simulink model "Oscillator_Sync_Aperiodic"  (Simulink 10.0)
settings: Solver=ode45  StartTime=0.0  StopTime=T  MaxStep=MaxStep  RelTol=RelTol  EnableMultiTasking=on
values from neighbouring files (symbols this model uses):
  J = 30    [initialization_Oscillator_Sync_Aperiodic.m]
  Kmatrix = [-1 -2]    [initialization_Oscillator_Sync_Aperiodic.m]
  rule = 1    [initialization_Oscillator_Sync_Aperiodic.m]
  T = 15    [initialization_Oscillator_Sync_Aperiodic.m]
undefined symbols (not defined in the file): x11_0, x1_0, x22_0, x2_0, x33_0, x3_0, x44_0, x4_0
libraries: simulink x24, HyEQ_Library_R2012a x2
(part 2 of 2)

== system Oscillator_Sync_Aperiodic/Aperiodic Sampling 4/Integrator System/Jump logic ==
  note: rule=1:  out = D
      | rlule=2: out = D and ~C
      | rule=3:  out = (D and ~C)  or (D and C and r>0.5)
      | other :  out = 0
  C : Inport
  D : Inport  Port=2
  r : Inport  Port=3
  Compare To Constant : simulink/Logic and Bit Operations/Compare To Constant  relop=>=  const=0.5  OutDataTypeStr=uint8
  Constant : Constant  Value=rule
  Logical Operator : Logic  AllPortsSameDT=off  OutDataTypeStr=boolean
  Logical Operator1 : Logic  Operator=NOT  Inputs=1  AllPortsSameDT=off  OutDataTypeStr=boolean
  Logical Operator2 : Logic  Operator=OR  AllPortsSameDT=off  OutDataTypeStr=boolean
  Logical Operator3 : Logic  Inputs=3  AllPortsSameDT=off  OutDataTypeStr=boolean
  Multiport Switch : MultiPortSwitch
  jump : Outport
  wires:
  Logical Operator3/1 -> Logical Operator2/2
  Compare To Constant/1 -> Logical Operator3/3
  Multiport Switch/1 -> jump/1
  Logical Operator2/1 -> Multiport Switch/4
  Logical Operator/1 -> Logical Operator2/1, Multiport Switch/3
  Logical Operator1/1 -> Logical Operator/2
  C/1 -> Logical Operator1/1, Logical Operator3/2
  r/1 -> Compare To Constant/1
  D/1 -> Multiport Switch/2, Logical Operator/1, Logical Operator3/1
  Constant/1 -> Multiport Switch/1

== system Oscillator_Sync_Aperiodic/Aperiodic Sampling 4/Integrator System/Stop logic ==
  t : Inport
  j : Inport  Port=2
  C : Inport  Port=3
  D : Inport  Port=4
  "Flow Horizon, T" : simulink/Logic and Bit Operations/Compare To Constant  relop=>=  const=T  OutDataTypeStr=uint8  ZeroCross=off
  "Jump Horizon, J" : simulink/Logic and Bit Operations/Compare To Constant  relop=>=  const=J  OutDataTypeStr=uint8  ZeroCross=off
  Logical Operator : Logic  Operator=NOR  AllPortsSameDT=off  OutDataTypeStr=boolean
  Logical Operator1 : Logic  Operator=OR  Inputs=3  AllPortsSameDT=off  OutDataTypeStr=boolean
  stop : Outport
  wires:
  Logical Operator1/1 -> stop/1
  C/1 -> Logical Operator/1
  j/1 -> "Jump Horizon, J"/1
  t/1 -> "Flow Horizon, T"/1
  D/1 -> Logical Operator/2
  Logical Operator/1 -> Logical Operator1/3
  "Jump Horizon, J"/1 -> Logical Operator1/2
  "Flow Horizon, T"/1 -> Logical Operator1/1

== system Oscillator_Sync_Aperiodic/Aperiodic Sampling 4/Integrator System/Update logic ==
  g(x-,u) : Inport
  j- : Inport  Port=2
  t- : Inport  Port=3
  Constant : Constant
  Mux1 : Mux  Inputs=[1 1 -1]
  Sum : Sum  Inputs=|++
  update law : Outport
  wires:
  Constant/1 -> Sum/2
  t-/1 -> Mux1/1
  g(x-,u)/1 -> Mux1/3
  j-/1 -> Sum/1
  Mux1/1 -> update law/1
  Sum/1 -> Mux1/2

== system Oscillator_Sync_Aperiodic/Oscillator 1/Integrator System/CT dynamics ==
  f(x,u) : Inport
  Flows : Constant
  Jumps : Constant  Value=0
  Mux : Mux  Inputs=[1 1 -1]
  dot : Outport
  wires:
  f(x,u)/1 -> Mux/3
  Mux/1 -> dot/1
  Flows/1 -> Mux/1
  Jumps/1 -> Mux/2

== system Oscillator_Sync_Aperiodic/Oscillator 1/Integrator System/Jump logic ==
  note: rule=1:  out = D
      | rlule=2: out = D and ~C
      | rule=3:  out = (D and ~C)  or (D and C and r>0.5)
      | other :  out = 0
  C : Inport
  D : Inport  Port=2
  r : Inport  Port=3
  Compare To Constant : simulink/Logic and Bit Operations/Compare To Constant  relop=>=  const=0.5  OutDataTypeStr=uint8
  Constant : Constant  Value=rule
  Logical Operator : Logic  AllPortsSameDT=off  OutDataTypeStr=boolean
  Logical Operator1 : Logic  Operator=NOT  Inputs=1  AllPortsSameDT=off  OutDataTypeStr=boolean
  Logical Operator2 : Logic  Operator=OR  AllPortsSameDT=off  OutDataTypeStr=boolean
  Logical Operator3 : Logic  Inputs=3  AllPortsSameDT=off  OutDataTypeStr=boolean
  Multiport Switch : MultiPortSwitch
  jump : Outport
  wires:
  Logical Operator3/1 -> Logical Operator2/2
  Compare To Constant/1 -> Logical Operator3/3
  Multiport Switch/1 -> jump/1
  Logical Operator2/1 -> Multiport Switch/4
  Logical Operator/1 -> Logical Operator2/1, Multiport Switch/3
  Logical Operator1/1 -> Logical Operator/2
  C/1 -> Logical Operator1/1, Logical Operator3/2
  r/1 -> Compare To Constant/1
  D/1 -> Multiport Switch/2, Logical Operator/1, Logical Operator3/1
  Constant/1 -> Multiport Switch/1

== system Oscillator_Sync_Aperiodic/Oscillator 1/Integrator System/Stop logic ==
  t : Inport
  j : Inport  Port=2
  C : Inport  Port=3
  D : Inport  Port=4
  "Flow Horizon, T" : simulink/Logic and Bit Operations/Compare To Constant  relop=>=  const=T  OutDataTypeStr=uint8  ZeroCross=off
  "Jump Horizon, J" : simulink/Logic and Bit Operations/Compare To Constant  relop=>=  const=J  OutDataTypeStr=uint8  ZeroCross=off
  Logical Operator : Logic  Operator=NOR  AllPortsSameDT=off  OutDataTypeStr=boolean
  Logical Operator1 : Logic  Operator=OR  Inputs=3  AllPortsSameDT=off  OutDataTypeStr=boolean
  stop : Outport
  wires:
  Logical Operator1/1 -> stop/1
  C/1 -> Logical Operator/1
  j/1 -> "Jump Horizon, J"/1
  t/1 -> "Flow Horizon, T"/1
  D/1 -> Logical Operator/2
  Logical Operator/1 -> Logical Operator1/3
  "Jump Horizon, J"/1 -> Logical Operator1/2
  "Flow Horizon, T"/1 -> Logical Operator1/1

== system Oscillator_Sync_Aperiodic/Oscillator 1/Integrator System/Update logic ==
  g(x-,u) : Inport
  j- : Inport  Port=2
  t- : Inport  Port=3
  Constant : Constant
  Mux1 : Mux  Inputs=[1 1 -1]
  Sum : Sum  Inputs=|++
  update law : Outport
  wires:
  Constant/1 -> Sum/2
  t-/1 -> Mux1/1
  g(x-,u)/1 -> Mux1/3
  j-/1 -> Sum/1
  Mux1/1 -> update law/1
  Sum/1 -> Mux1/2

== system Oscillator_Sync_Aperiodic/Oscillator 2/Integrator System/CT dynamics ==
  f(x,u) : Inport
  Flows : Constant
  Jumps : Constant  Value=0
  Mux : Mux  Inputs=[1 1 -1]
  dot : Outport
  wires:
  f(x,u)/1 -> Mux/3
  Mux/1 -> dot/1
  Flows/1 -> Mux/1
  Jumps/1 -> Mux/2

== system Oscillator_Sync_Aperiodic/Oscillator 2/Integrator System/Jump logic ==
  note: rule=1:  out = D
      | rlule=2: out = D and ~C
      | rule=3:  out = (D and ~C)  or (D and C and r>0.5)
      | other :  out = 0
  C : Inport
  D : Inport  Port=2
  r : Inport  Port=3
  Compare To Constant : simulink/Logic and Bit Operations/Compare To Constant  relop=>=  const=0.5  OutDataTypeStr=uint8
  Constant : Constant  Value=rule
  Logical Operator : Logic  AllPortsSameDT=off  OutDataTypeStr=boolean
  Logical Operator1 : Logic  Operator=NOT  Inputs=1  AllPortsSameDT=off  OutDataTypeStr=boolean
  Logical Operator2 : Logic  Operator=OR  AllPortsSameDT=off  OutDataTypeStr=boolean
  Logical Operator3 : Logic  Inputs=3  AllPortsSameDT=off  OutDataTypeStr=boolean
  Multiport Switch : MultiPortSwitch
  jump : Outport
  wires:
  Logical Operator3/1 -> Logical Operator2/2
  Compare To Constant/1 -> Logical Operator3/3
  Multiport Switch/1 -> jump/1
  Logical Operator2/1 -> Multiport Switch/4
  Logical Operator/1 -> Logical Operator2/1, Multiport Switch/3
  Logical Operator1/1 -> Logical Operator/2
  C/1 -> Logical Operator1/1, Logical Operator3/2
  r/1 -> Compare To Constant/1
  D/1 -> Multiport Switch/2, Logical Operator/1, Logical Operator3/1
  Constant/1 -> Multiport Switch/1

== system Oscillator_Sync_Aperiodic/Oscillator 2/Integrator System/Stop logic ==
  t : Inport
  j : Inport  Port=2
  C : Inport  Port=3
  D : Inport  Port=4
  "Flow Horizon, T" : simulink/Logic and Bit Operations/Compare To Constant  relop=>=  const=T  OutDataTypeStr=uint8  ZeroCross=off
  "Jump Horizon, J" : simulink/Logic and Bit Operations/Compare To Constant  relop=>=  const=J  OutDataTypeStr=uint8  ZeroCross=off
  Logical Operator : Logic  Operator=NOR  AllPortsSameDT=off  OutDataTypeStr=boolean
  Logical Operator1 : Logic  Operator=OR  Inputs=3  AllPortsSameDT=off  OutDataTypeStr=boolean
  stop : Outport
  wires:
  Logical Operator1/1 -> stop/1
  C/1 -> Logical Operator/1
  j/1 -> "Jump Horizon, J"/1
  t/1 -> "Flow Horizon, T"/1
  D/1 -> Logical Operator/2
  Logical Operator/1 -> Logical Operator1/3
  "Jump Horizon, J"/1 -> Logical Operator1/2
  "Flow Horizon, T"/1 -> Logical Operator1/1

== system Oscillator_Sync_Aperiodic/Oscillator 2/Integrator System/Update logic ==
  g(x-,u) : Inport
  j- : Inport  Port=2
  t- : Inport  Port=3
  Constant : Constant
  Mux1 : Mux  Inputs=[1 1 -1]
  Sum : Sum  Inputs=|++
  update law : Outport
  wires:
  Constant/1 -> Sum/2
  t-/1 -> Mux1/1
  g(x-,u)/1 -> Mux1/3
  j-/1 -> Sum/1
  Mux1/1 -> update law/1
  Sum/1 -> Mux1/2

== system Oscillator_Sync_Aperiodic/Oscillator 3/Integrator System/CT dynamics ==
  f(x,u) : Inport
  Flows : Constant
  Jumps : Constant  Value=0
  Mux : Mux  Inputs=[1 1 -1]
  dot : Outport
  wires:
  f(x,u)/1 -> Mux/3
  Mux/1 -> dot/1
  Flows/1 -> Mux/1
  Jumps/1 -> Mux/2

== system Oscillator_Sync_Aperiodic/Oscillator 3/Integrator System/Jump logic ==
  note: rule=1:  out = D
      | rlule=2: out = D and ~C
      | rule=3:  out = (D and ~C)  or (D and C and r>0.5)
      | other :  out = 0
  C : Inport
  D : Inport  Port=2
  r : Inport  Port=3
  Compare To Constant : simulink/Logic and Bit Operations/Compare To Constant  relop=>=  const=0.5  OutDataTypeStr=uint8
  Constant : Constant  Value=rule
  Logical Operator : Logic  AllPortsSameDT=off  OutDataTypeStr=boolean
  Logical Operator1 : Logic  Operator=NOT  Inputs=1  AllPortsSameDT=off  OutDataTypeStr=boolean
  Logical Operator2 : Logic  Operator=OR  AllPortsSameDT=off  OutDataTypeStr=boolean
  Logical Operator3 : Logic  Inputs=3  AllPortsSameDT=off  OutDataTypeStr=boolean
  Multiport Switch : MultiPortSwitch
  jump : Outport
  wires:
  Logical Operator3/1 -> Logical Operator2/2
  Compare To Constant/1 -> Logical Operator3/3
  Multiport Switch/1 -> jump/1
  Logical Operator2/1 -> Multiport Switch/4
  Logical Operator/1 -> Logical Operator2/1, Multiport Switch/3
  Logical Operator1/1 -> Logical Operator/2
  C/1 -> Logical Operator1/1, Logical Operator3/2
  r/1 -> Compare To Constant/1
  D/1 -> Multiport Switch/2, Logical Operator/1, Logical Operator3/1
  Constant/1 -> Multiport Switch/1

== system Oscillator_Sync_Aperiodic/Oscillator 3/Integrator System/Stop logic ==
  t : Inport
  j : Inport  Port=2
  C : Inport  Port=3
  D : Inport  Port=4
  "Flow Horizon, T" : simulink/Logic and Bit Operations/Compare To Constant  relop=>=  const=T  OutDataTypeStr=uint8  ZeroCross=off
  "Jump Horizon, J" : simulink/Logic and Bit Operations/Compare To Constant  relop=>=  const=J  OutDataTypeStr=uint8  ZeroCross=off
  Logical Operator : Logic  Operator=NOR  AllPortsSameDT=off  OutDataTypeStr=boolean
  Logical Operator1 : Logic  Operator=OR  Inputs=3  AllPortsSameDT=off  OutDataTypeStr=boolean
  stop : Outport
  wires:
  Logical Operator1/1 -> stop/1
  C/1 -> Logical Operator/1
  j/1 -> "Jump Horizon, J"/1
  t/1 -> "Flow Horizon, T"/1
  D/1 -> Logical Operator/2
  Logical Operator/1 -> Logical Operator1/3
  "Jump Horizon, J"/1 -> Logical Operator1/2
  "Flow Horizon, T"/1 -> Logical Operator1/1

== system Oscillator_Sync_Aperiodic/Oscillator 3/Integrator System/Update logic ==
  g(x-,u) : Inport
  j- : Inport  Port=2
  t- : Inport  Port=3
  Constant : Constant
  Mux1 : Mux  Inputs=[1 1 -1]
  Sum : Sum  Inputs=|++
  update law : Outport
  wires:
  Constant/1 -> Sum/2
  t-/1 -> Mux1/1
  g(x-,u)/1 -> Mux1/3
  j-/1 -> Sum/1
  Mux1/1 -> update law/1
  Sum/1 -> Mux1/2

== system Oscillator_Sync_Aperiodic/Oscillator 4/Integrator System/CT dynamics ==
  f(x,u) : Inport
  Flows : Constant
  Jumps : Constant  Value=0
  Mux : Mux  Inputs=[1 1 -1]
  dot : Outport
  wires:
  f(x,u)/1 -> Mux/3
  Mux/1 -> dot/1
  Flows/1 -> Mux/1
  Jumps/1 -> Mux/2

== system Oscillator_Sync_Aperiodic/Oscillator 4/Integrator System/Jump logic ==
  note: rule=1:  out = D
      | rlule=2: out = D and ~C
      | rule=3:  out = (D and ~C)  or (D and C and r>0.5)
      | other :  out = 0
  C : Inport
  D : Inport  Port=2
  r : Inport  Port=3
  Compare To Constant : simulink/Logic and Bit Operations/Compare To Constant  relop=>=  const=0.5  OutDataTypeStr=uint8
  Constant : Constant  Value=rule
  Logical Operator : Logic  AllPortsSameDT=off  OutDataTypeStr=boolean
  Logical Operator1 : Logic  Operator=NOT  Inputs=1  AllPortsSameDT=off  OutDataTypeStr=boolean
  Logical Operator2 : Logic  Operator=OR  AllPortsSameDT=off  OutDataTypeStr=boolean
  Logical Operator3 : Logic  Inputs=3  AllPortsSameDT=off  OutDataTypeStr=boolean
  Multiport Switch : MultiPortSwitch
  jump : Outport
  wires:
  Logical Operator3/1 -> Logical Operator2/2
  Compare To Constant/1 -> Logical Operator3/3
  Multiport Switch/1 -> jump/1
  Logical Operator2/1 -> Multiport Switch/4
  Logical Operator/1 -> Logical Operator2/1, Multiport Switch/3
  Logical Operator1/1 -> Logical Operator/2
  C/1 -> Logical Operator1/1, Logical Operator3/2
  r/1 -> Compare To Constant/1
  D/1 -> Multiport Switch/2, Logical Operator/1, Logical Operator3/1
  Constant/1 -> Multiport Switch/1

== system Oscillator_Sync_Aperiodic/Oscillator 4/Integrator System/Stop logic ==
  t : Inport
  j : Inport  Port=2
  C : Inport  Port=3
  D : Inport  Port=4
  "Flow Horizon, T" : simulink/Logic and Bit Operations/Compare To Constant  relop=>=  const=T  OutDataTypeStr=uint8  ZeroCross=off
  "Jump Horizon, J" : simulink/Logic and Bit Operations/Compare To Constant  relop=>=  const=J  OutDataTypeStr=uint8  ZeroCross=off
  Logical Operator : Logic  Operator=NOR  AllPortsSameDT=off  OutDataTypeStr=boolean
  Logical Operator1 : Logic  Operator=OR  Inputs=3  AllPortsSameDT=off  OutDataTypeStr=boolean
  stop : Outport
  wires:
  Logical Operator1/1 -> stop/1
  C/1 -> Logical Operator/1
  j/1 -> "Jump Horizon, J"/1
  t/1 -> "Flow Horizon, T"/1
  D/1 -> Logical Operator/2
  Logical Operator/1 -> Logical Operator1/3
  "Jump Horizon, J"/1 -> Logical Operator1/2
  "Flow Horizon, T"/1 -> Logical Operator1/1

== system Oscillator_Sync_Aperiodic/Oscillator 4/Integrator System/Update logic ==
  g(x-,u) : Inport
  j- : Inport  Port=2
  t- : Inport  Port=3
  Constant : Constant
  Mux1 : Mux  Inputs=[1 1 -1]
  Sum : Sum  Inputs=|++
  update law : Outport
  wires:
  Constant/1 -> Sum/2
  t-/1 -> Mux1/1
  g(x-,u)/1 -> Mux1/3
  j-/1 -> Sum/1
  Mux1/1 -> update law/1
  Sum/1 -> Mux1/2

== matlab function Oscillator 1/flow map f ==
  data: tau input double; taudot output double; u input double
function taudot = f(tau, u)

%%%%%%%%%%%%%%%%%%%%%%%%%%%%%%%%%%%%%%%%%%%%%%%%%%%%%%%%%%%%%%%%%%%%%%%%%%%
% Matlab Function  Author: Ricardo Sanfelice
%
% Project: Simulation of a hybrid system (interconnection)
%
% Name: f.m
%
% Description: Flow map
%
% Version: 1.0
% Required files: - 
%%%%%%%%%%%%%%%%%%%%%%%%%%%%%%%%%%%%%%%%%%%%%%%%%%%%%%%%%%%%%%%%%%%%%%%%%%%

% flow map
Amatrix = [0 1;-1 0];
Bmatrix = [0;1];
taudot = Amatrix*tau + Bmatrix*u;

== matlab function Oscillator 1/flow set C ==
  data: tau input double; v output double; u input double
function v  = C(tau, u) 

%%%%%%%%%%%%%%%%%%%%%%%%%%%%%%%%%%%%%%%%%%%%%%%%%%%%%%%%%%%%%%%%%%%%%%%%%%%
% Matlab Function  Author: Ricardo Sanfelice 
%
% Project: Simulation of a hybrid system (interconnection)
%
% Name: C.m
%
% Description: Flow set
%
% Version: 1.0
% Required files: - 
%%%%%%%%%%%%%%%%%%%%%%%%%%%%%%%%%%%%%%%%%%%%%%%%%%%%%%%%%%%%%%%%%%%%%%%%%%%

%flow set
% if ((tau > 0) && (tau < 1)) || ((u > 0) && (u <= 1))  % flow condition
%     v = 1;  % report flow
% else 
%     v = 0;  % do not report flow
% end
v = 1;

== matlab function Oscillator 2/flow map f ==
  data: tau input double; taudot output double; u input double
function taudot = f(tau, u)

%%%%%%%%%%%%%%%%%%%%%%%%%%%%%%%%%%%%%%%%%%%%%%%%%%%%%%%%%%%%%%%%%%%%%%%%%%%
% Matlab Function  Author: Ricardo Sanfelice
%
% Project: Simulation of a hybrid system (interconnection)
%
% Name: f.m
%
% Description: Flow map
%
% Version: 1.0
% Required files: - 
%%%%%%%%%%%%%%%%%%%%%%%%%%%%%%%%%%%%%%%%%%%%%%%%%%%%%%%%%%%%%%%%%%%%%%%%%%%

% flow map
Amatrix = [0 1;-1 0];
Bmatrix = [0;1];
taudot = Amatrix*tau + Bmatrix*u;

== matlab function Oscillator 2/flow set C ==
  data: tau input double; v output double; u input double
function v  = C(tau, u) 

%%%%%%%%%%%%%%%%%%%%%%%%%%%%%%%%%%%%%%%%%%%%%%%%%%%%%%%%%%%%%%%%%%%%%%%%%%%
% Matlab Function  Author: Ricardo Sanfelice 
%
% Project: Simulation of a hybrid system (interconnection)
%
% Name: C.m
%
% Description: Flow set
%
% Version: 1.0
% Required files: - 
%%%%%%%%%%%%%%%%%%%%%%%%%%%%%%%%%%%%%%%%%%%%%%%%%%%%%%%%%%%%%%%%%%%%%%%%%%%

%flow set
% if ((tau > 0) && (tau < 1)) || ((u > 0) && (u <= 1))  % flow condition
%     v = 1;  % report flow
% else 
%     v = 0;  % do not report flow
% end
v = 1;

== matlab function Oscillator 2/jump map g ==
  data: tau input double; tauplus output double; u input double
function tauplus = g(tau, u)

%%%%%%%%%%%%%%%%%%%%%%%%%%%%%%%%%%%%%%%%%%%%%%%%%%%%%%%%%%%%%%%%%%%%%%%%%%%
% Matlab Function  Author: Ricardo Sanfelice 
%
% Project: Simulation of a hybrid system (interconnection)
%
% Name: g.m
%
% Description: Jump map
%
% Version: 1.0
% Required files: - 
%%%%%%%%%%%%%%%%%%%%%%%%%%%%%%%%%%%%%%%%%%%%%%%%%%%%%%%%%%%%%%%%%%%%%%%%%%%

% jump map
% if (1+e)*tau < 1
%     tauplus = (1+e)*tau;
% elseif (1+e)*tau >= 1
%     tauplus = 0;
% else
%     tauplus = tau;   
% end
tauplus = [1;0];

== matlab function Oscillator 1/jump map g ==
  data: tau input double; tauplus output double; u input double
function tauplus = g(tau, u)

%%%%%%%%%%%%%%%%%%%%%%%%%%%%%%%%%%%%%%%%%%%%%%%%%%%%%%%%%%%%%%%%%%%%%%%%%%%
% Matlab Function  Author: Ricardo Sanfelice 
%
% Project: Simulation of a hybrid system (interconnection)
%
% Name: g.m
%
% Description: Jump map
%
% Version: 1.0
% Required files: - 
%%%%%%%%%%%%%%%%%%%%%%%%%%%%%%%%%%%%%%%%%%%%%%%%%%%%%%%%%%%%%%%%%%%%%%%%%%%

% jump map
% if (1+e)*tau < 1
%     tauplus = (1+e)*tau;
% elseif (1+e)*tau >= 1
%     tauplus = 0;
% else
%     tauplus = tau;   
% end
tauplus = [-1;0];

== matlab function Oscillator 1/jump set D ==
  data: tau input double; v output double; u input double
function v  = D(tau, u) 

%%%%%%%%%%%%%%%%%%%%%%%%%%%%%%%%%%%%%%%%%%%%%%%%%%%%%%%%%%%%%%%%%%%%%%%%%%%
% Matlab Function  Author: Ricardo Sanfelice
%
% Project: Simulation of a hybrid system (interconnection)
%
% Name: D.m
%
% Description: Jump set
%
% Version: 1.0
% Required files: - 
%%%%%%%%%%%%%%%%%%%%%%%%%%%%%%%%%%%%%%%%%%%%%%%%%%%%%%%%%%%%%%%%%%%%%%%%%%%

% if (u >= 1) || (tau >= 1) % jump condition
%     v = 1;  % report jump
% else
%     v = 0;  % do not report jump
% end
v = 0;

== matlab function Oscillator 2/jump set D ==
  data: tau input double; v output double; u input double
function v  = D(tau, u) 

%%%%%%%%%%%%%%%%%%%%%%%%%%%%%%%%%%%%%%%%%%%%%%%%%%%%%%%%%%%%%%%%%%%%%%%%%%%
% Matlab Function  Author: Ricardo Sanfelice
%
% Project: Simulation of a hybrid system (interconnection)
%
% Name: D.m
%
% Description: Jump set
%
% Version: 1.0
% Required files: - 
%%%%%%%%%%%%%%%%%%%%%%%%%%%%%%%%%%%%%%%%%%%%%%%%%%%%%%%%%%%%%%%%%%%%%%%%%%%

% if (u >= 1) || (tau >= 1) % jump condition
%     v = 1;  % report jump
% else
%     v = 0;  % do not report jump
% end
v = 0;

== matlab function Oscillator 3/flow map f ==
  data: tau input double; taudot output double; u input double
function taudot = f(tau, u)

%%%%%%%%%%%%%%%%%%%%%%%%%%%%%%%%%%%%%%%%%%%%%%%%%%%%%%%%%%%%%%%%%%%%%%%%%%%
% Matlab Function  Author: Ricardo Sanfelice
%
% Project: Simulation of a hybrid system (interconnection)
%
% Name: f.m
%
% Description: Flow map
%
% Version: 1.0
% Required files: - 
%%%%%%%%%%%%%%%%%%%%%%%%%%%%%%%%%%%%%%%%%%%%%%%%%%%%%%%%%%%%%%%%%%%%%%%%%%%

% flow map
Amatrix = [0 1;-1 0];
Bmatrix = [0;1];
taudot = Amatrix*tau + Bmatrix*u;

== matlab function Oscillator 3/flow set C ==
  data: tau input double; v output double; u input double
function v  = C(tau, u) 

%%%%%%%%%%%%%%%%%%%%%%%%%%%%%%%%%%%%%%%%%%%%%%%%%%%%%%%%%%%%%%%%%%%%%%%%%%%
% Matlab Function  Author: Ricardo Sanfelice 
%
% Project: Simulation of a hybrid system (interconnection)
%
% Name: C.m
%
% Description: Flow set
%
% Version: 1.0
% Required files: - 
%%%%%%%%%%%%%%%%%%%%%%%%%%%%%%%%%%%%%%%%%%%%%%%%%%%%%%%%%%%%%%%%%%%%%%%%%%%

%flow set
% if ((tau > 0) && (tau < 1)) || ((u > 0) && (u <= 1))  % flow condition
%     v = 1;  % report flow
% else 
%     v = 0;  % do not report flow
% end
v = 1;

== matlab function Oscillator 3/jump map g ==
  data: tau input double; tauplus output double; u input double
function tauplus = g(tau, u)

%%%%%%%%%%%%%%%%%%%%%%%%%%%%%%%%%%%%%%%%%%%%%%%%%%%%%%%%%%%%%%%%%%%%%%%%%%%
% Matlab Function  Author: Ricardo Sanfelice 
%
% Project: Simulation of a hybrid system (interconnection)
%
% Name: g.m
%
% Description: Jump map
%
% Version: 1.0
% Required files: - 
%%%%%%%%%%%%%%%%%%%%%%%%%%%%%%%%%%%%%%%%%%%%%%%%%%%%%%%%%%%%%%%%%%%%%%%%%%%

% jump map
% if (1+e)*tau < 1
%     tauplus = (1+e)*tau;
% elseif (1+e)*tau >= 1
%     tauplus = 0;
% else
%     tauplus = tau;   
% end
tauplus = [0.5;0];

== matlab function Oscillator 3/jump set D ==
  data: tau input double; v output double; u input double
function v  = D(tau, u) 

%%%%%%%%%%%%%%%%%%%%%%%%%%%%%%%%%%%%%%%%%%%%%%%%%%%%%%%%%%%%%%%%%%%%%%%%%%%
% Matlab Function  Author: Ricardo Sanfelice
%
% Project: Simulation of a hybrid system (interconnection)
%
% Name: D.m
%
% Description: Jump set
%
% Version: 1.0
% Required files: - 
%%%%%%%%%%%%%%%%%%%%%%%%%%%%%%%%%%%%%%%%%%%%%%%%%%%%%%%%%%%%%%%%%%%%%%%%%%%

% if (u >= 1) || (tau >= 1) % jump condition
%     v = 1;  % report jump
% else
%     v = 0;  % do not report jump
% end
v = 0;

== matlab function Oscillator 4/flow map f ==
  data: tau input double; taudot output double; u input double
function taudot = f(tau, u)

%%%%%%%%%%%%%%%%%%%%%%%%%%%%%%%%%%%%%%%%%%%%%%%%%%%%%%%%%%%%%%%%%%%%%%%%%%%
% Matlab Function  Author: Ricardo Sanfelice
%
% Project: Simulation of a hybrid system (interconnection)
%
% Name: f.m
%
% Description: Flow map
%
% Version: 1.0
% Required files: - 
%%%%%%%%%%%%%%%%%%%%%%%%%%%%%%%%%%%%%%%%%%%%%%%%%%%%%%%%%%%%%%%%%%%%%%%%%%%

% flow map
Amatrix = [0 1;-1 0];
Bmatrix = [0;1];
taudot = Amatrix*tau + Bmatrix*u;

== matlab function Oscillator 4/flow set C ==
  data: tau input double; v output double; u input double
function v  = C(tau, u) 

%%%%%%%%%%%%%%%%%%%%%%%%%%%%%%%%%%%%%%%%%%%%%%%%%%%%%%%%%%%%%%%%%%%%%%%%%%%
% Matlab Function  Author: Ricardo Sanfelice 
%
% Project: Simulation of a hybrid system (interconnection)
%
% Name: C.m
%
% Description: Flow set
%
% Version: 1.0
% Required files: - 
%%%%%%%%%%%%%%%%%%%%%%%%%%%%%%%%%%%%%%%%%%%%%%%%%%%%%%%%%%%%%%%%%%%%%%%%%%%

%flow set
% if ((tau > 0) && (tau < 1)) || ((u > 0) && (u <= 1))  % flow condition
%     v = 1;  % report flow
% else 
%     v = 0;  % do not report flow
% end
v = 1;

== matlab function Oscillator 4/jump map g ==
  data: tau input double; tauplus output double; u input double
function tauplus = g(tau, u)

%%%%%%%%%%%%%%%%%%%%%%%%%%%%%%%%%%%%%%%%%%%%%%%%%%%%%%%%%%%%%%%%%%%%%%%%%%%
% Matlab Function  Author: Ricardo Sanfelice 
%
% Project: Simulation of a hybrid system (interconnection)
%
% Name: g.m
%
% Description: Jump map
%
% Version: 1.0
% Required files: - 
%%%%%%%%%%%%%%%%%%%%%%%%%%%%%%%%%%%%%%%%%%%%%%%%%%%%%%%%%%%%%%%%%%%%%%%%%%%

% jump map
% if (1+e)*tau < 1
%     tauplus = (1+e)*tau;
% elseif (1+e)*tau >= 1
%     tauplus = 0;
% else
%     tauplus = tau;   
% end
tauplus = [2;0];

== matlab function Oscillator 4/jump set D ==
  data: tau input double; v output double; u input double
function v  = D(tau, u) 

%%%%%%%%%%%%%%%%%%%%%%%%%%%%%%%%%%%%%%%%%%%%%%%%%%%%%%%%%%%%%%%%%%%%%%%%%%%
% Matlab Function  Author: Ricardo Sanfelice
%
% Project: Simulation of a hybrid system (interconnection)
%
% Name: D.m
%
% Description: Jump set
%
% Version: 1.0
% Required files: - 
%%%%%%%%%%%%%%%%%%%%%%%%%%%%%%%%%%%%%%%%%%%%%%%%%%%%%%%%%%%%%%%%%%%%%%%%%%%

% if (u >= 1) || (tau >= 1) % jump condition
%     v = 1;  % report jump
% else
%     v = 0;  % do not report jump
% end
v = 0;

== matlab function Aperiodic Sampling 1/flow map f ==
  data: tau input double; taudot output double; u input double
function taudot = f(tau, u)

%%%%%%%%%%%%%%%%%%%%%%%%%%%%%%%%%%%%%%%%%%%%%%%%%%%%%%%%%%%%%%%%%%%%%%%%%%%
% Matlab Function  Author: Ricardo Sanfelice
%
% Project: Simulation of a hybrid system (interconnection)
%
% Name: f.m
%
% Description: Flow map
%
% Version: 1.0
% Required files: - 
%%%%%%%%%%%%%%%%%%%%%%%%%%%%%%%%%%%%%%%%%%%%%%%%%%%%%%%%%%%%%%%%%%%%%%%%%%%

% flow map
taudot = [0;1;0];

== matlab function Aperiodic Sampling 1/flow set C ==
  data: tau input double; v output double; u input double
function v  = C(tau, u) 

%%%%%%%%%%%%%%%%%%%%%%%%%%%%%%%%%%%%%%%%%%%%%%%%%%%%%%%%%%%%%%%%%%%%%%%%%%%
% Matlab Function  Author: Ricardo Sanfelice 
%
% Project: Simulation of a hybrid system (interconnection)
%
% Name: C.m
%
% Description: Flow set
%
% Version: 1.0
% Required files: - 
%%%%%%%%%%%%%%%%%%%%%%%%%%%%%%%%%%%%%%%%%%%%%%%%%%%%%%%%%%%%%%%%%%%%%%%%%%%

%flow set
if ((tau(2) >= 0) && (tau(2) < tau(3)))   % flow condition
    v = 1;  % report flow
else 
    v = 0;  % do not report flow
end

== matlab function Aperiodic Sampling 1/jump map g ==
  settings: updateMethod=DISCRETE
  data: tau input double; tauplus output double; u input double
function tauplus = g(tau, u)

%%%%%%%%%%%%%%%%%%%%%%%%%%%%%%%%%%%%%%%%%%%%%%%%%%%%%%%%%%%%%%%%%%%%%%%%%%%
% Matlab Function  Author: Ricardo Sanfelice 
%
% Project: Simulation of a hybrid system (interconnection)
%
% Name: g.m
%
% Description: Jump map
%
% Version: 1.0
% Required files: - 
%%%%%%%%%%%%%%%%%%%%%%%%%%%%%%%%%%%%%%%%%%%%%%%%%%%%%%%%%%%%%%%%%%%%%%%%%%%

% jump map
% if (1+e)*tau < 1
%     tauplus = (1+e)*tau;
% elseif (1+e)*tau >= 1
%     tauplus = 0;
% else
%     tauplus = tau;   
% end
tauplus = zeros(3,1);
tauplus(1) = u;
tauplus(2) = 0;
tauplus(3) = 0.3+0.35*rand;

== matlab function Aperiodic Sampling 1/jump set D ==
  data: tau input double; v output double; u input double
function v  = D(tau, u) 

%%%%%%%%%%%%%%%%%%%%%%%%%%%%%%%%%%%%%%%%%%%%%%%%%%%%%%%%%%%%%%%%%%%%%%%%%%%
% Matlab Function  Author: Ricardo Sanfelice
%
% Project: Simulation of a hybrid system (interconnection)
%
% Name: D.m
%
% Description: Jump set
%
% Version: 1.0
% Required files: - 
%%%%%%%%%%%%%%%%%%%%%%%%%%%%%%%%%%%%%%%%%%%%%%%%%%%%%%%%%%%%%%%%%%%%%%%%%%%

if (tau(2) >= tau(3)) % jump condition
    v = 1;  % report jump
else
    v = 0;  % do not report jump
end

== matlab function Aperiodic Sampling 2/flow map f ==
  data: tau input double; taudot output double; u input double
function taudot = f(tau, u)

%%%%%%%%%%%%%%%%%%%%%%%%%%%%%%%%%%%%%%%%%%%%%%%%%%%%%%%%%%%%%%%%%%%%%%%%%%%
% Matlab Function  Author: Ricardo Sanfelice
%
% Project: Simulation of a hybrid system (interconnection)
%
% Name: f.m
%
% Description: Flow map
%
% Version: 1.0
% Required files: - 
%%%%%%%%%%%%%%%%%%%%%%%%%%%%%%%%%%%%%%%%%%%%%%%%%%%%%%%%%%%%%%%%%%%%%%%%%%%

% flow map
taudot = [0;1;0];

== matlab function Aperiodic Sampling 2/flow set C ==
  data: tau input double; v output double; u input double
function v  = C(tau, u) 

%%%%%%%%%%%%%%%%%%%%%%%%%%%%%%%%%%%%%%%%%%%%%%%%%%%%%%%%%%%%%%%%%%%%%%%%%%%
% Matlab Function  Author: Ricardo Sanfelice 
%
% Project: Simulation of a hybrid system (interconnection)
%
% Name: C.m
%
% Description: Flow set
%
% Version: 1.0
% Required files: - 
%%%%%%%%%%%%%%%%%%%%%%%%%%%%%%%%%%%%%%%%%%%%%%%%%%%%%%%%%%%%%%%%%%%%%%%%%%%

%flow set
if ((tau(2) >= 0) && (tau(2) < tau(3)))   % flow condition
    v = 1;  % report flow
else 
    v = 0;  % do not report flow
end

== matlab function Aperiodic Sampling 2/jump map g ==
  settings: updateMethod=DISCRETE
  data: tau input double; tauplus output double; u input double
function tauplus = g(tau, u)

%%%%%%%%%%%%%%%%%%%%%%%%%%%%%%%%%%%%%%%%%%%%%%%%%%%%%%%%%%%%%%%%%%%%%%%%%%%
% Matlab Function  Author: Ricardo Sanfelice 
%
% Project: Simulation of a hybrid system (interconnection)
%
% Name: g.m
%
% Description: Jump map
%
% Version: 1.0
% Required files: - 
%%%%%%%%%%%%%%%%%%%%%%%%%%%%%%%%%%%%%%%%%%%%%%%%%%%%%%%%%%%%%%%%%%%%%%%%%%%

% jump map
% if (1+e)*tau < 1
%     tauplus = (1+e)*tau;
% elseif (1+e)*tau >= 1
%     tauplus = 0;
% else
%     tauplus = tau;   
% end
tauplus = zeros(3,1);
tauplus(1) = u;
tauplus(2) = 0;
tauplus(3) = 0.3+0.35*rand;

== matlab function Aperiodic Sampling 2/jump set D ==
  data: tau input double; v output double; u input double
function v  = D(tau, u) 

%%%%%%%%%%%%%%%%%%%%%%%%%%%%%%%%%%%%%%%%%%%%%%%%%%%%%%%%%%%%%%%%%%%%%%%%%%%
% Matlab Function  Author: Ricardo Sanfelice
%
% Project: Simulation of a hybrid system (interconnection)
%
% Name: D.m
%
% Description: Jump set
%
% Version: 1.0
% Required files: - 
%%%%%%%%%%%%%%%%%%%%%%%%%%%%%%%%%%%%%%%%%%%%%%%%%%%%%%%%%%%%%%%%%%%%%%%%%%%

if (tau(2) >= tau(3)) % jump condition
    v = 1;  % report jump
else
    v = 0;  % do not report jump
end

== matlab function Aperiodic Sampling 3/flow map f ==
  data: tau input double; taudot output double; u input double
function taudot = f(tau, u)

%%%%%%%%%%%%%%%%%%%%%%%%%%%%%%%%%%%%%%%%%%%%%%%%%%%%%%%%%%%%%%%%%%%%%%%%%%%
% Matlab Function  Author: Ricardo Sanfelice
%
% Project: Simulation of a hybrid system (interconnection)
%
% Name: f.m
%
% Description: Flow map
%
% Version: 1.0
% Required files: - 
%%%%%%%%%%%%%%%%%%%%%%%%%%%%%%%%%%%%%%%%%%%%%%%%%%%%%%%%%%%%%%%%%%%%%%%%%%%

% flow map
taudot = [0;1;0];

== matlab function Aperiodic Sampling 3/flow set C ==
  data: tau input double; v output double; u input double
function v  = C(tau, u) 

%%%%%%%%%%%%%%%%%%%%%%%%%%%%%%%%%%%%%%%%%%%%%%%%%%%%%%%%%%%%%%%%%%%%%%%%%%%
% Matlab Function  Author: Ricardo Sanfelice 
%
% Project: Simulation of a hybrid system (interconnection)
%
% Name: C.m
%
% Description: Flow set
%
% Version: 1.0
% Required files: - 
%%%%%%%%%%%%%%%%%%%%%%%%%%%%%%%%%%%%%%%%%%%%%%%%%%%%%%%%%%%%%%%%%%%%%%%%%%%

%flow set
if ((tau(2) >= 0) && (tau(2) < tau(3)))   % flow condition
    v = 1;  % report flow
else 
    v = 0;  % do not report flow
end

== matlab function Aperiodic Sampling 3/jump map g ==
  settings: updateMethod=DISCRETE
  data: tau input double; tauplus output double; u input double
function tauplus = g(tau, u)

%%%%%%%%%%%%%%%%%%%%%%%%%%%%%%%%%%%%%%%%%%%%%%%%%%%%%%%%%%%%%%%%%%%%%%%%%%%
% Matlab Function  Author: Ricardo Sanfelice 
%
% Project: Simulation of a hybrid system (interconnection)
%
% Name: g.m
%
% Description: Jump map
%
% Version: 1.0
% Required files: - 
%%%%%%%%%%%%%%%%%%%%%%%%%%%%%%%%%%%%%%%%%%%%%%%%%%%%%%%%%%%%%%%%%%%%%%%%%%%

% jump map
% if (1+e)*tau < 1
%     tauplus = (1+e)*tau;
% elseif (1+e)*tau >= 1
%     tauplus = 0;
% else
%     tauplus = tau;   
% end
tauplus = zeros(3,1);
tauplus(1) = u;
tauplus(2) = 0;
tauplus(3) = 0.3+0.35*rand;

== matlab function Aperiodic Sampling 3/jump set D ==
  data: tau input double; v output double; u input double
function v  = D(tau, u) 

%%%%%%%%%%%%%%%%%%%%%%%%%%%%%%%%%%%%%%%%%%%%%%%%%%%%%%%%%%%%%%%%%%%%%%%%%%%
% Matlab Function  Author: Ricardo Sanfelice
%
% Project: Simulation of a hybrid system (interconnection)
%
% Name: D.m
%
% Description: Jump set
%
% Version: 1.0
% Required files: - 
%%%%%%%%%%%%%%%%%%%%%%%%%%%%%%%%%%%%%%%%%%%%%%%%%%%%%%%%%%%%%%%%%%%%%%%%%%%

if (tau(2) >= tau(3)) % jump condition
    v = 1;  % report jump
else
    v = 0;  % do not report jump
end

== matlab function Aperiodic Sampling 4/flow map f ==
  data: tau input double; taudot output double; u input double
function taudot = f(tau, u)

%%%%%%%%%%%%%%%%%%%%%%%%%%%%%%%%%%%%%%%%%%%%%%%%%%%%%%%%%%%%%%%%%%%%%%%%%%%
% Matlab Function  Author: Ricardo Sanfelice
%
% Project: Simulation of a hybrid system (interconnection)
%
% Name: f.m
%
% Description: Flow map
%
% Version: 1.0
% Required files: - 
%%%%%%%%%%%%%%%%%%%%%%%%%%%%%%%%%%%%%%%%%%%%%%%%%%%%%%%%%%%%%%%%%%%%%%%%%%%

% flow map
taudot = [0;1;0];

== matlab function Aperiodic Sampling 4/flow set C ==
  data: tau input double; v output double; u input double
function v  = C(tau, u) 

%%%%%%%%%%%%%%%%%%%%%%%%%%%%%%%%%%%%%%%%%%%%%%%%%%%%%%%%%%%%%%%%%%%%%%%%%%%
% Matlab Function  Author: Ricardo Sanfelice 
%
% Project: Simulation of a hybrid system (interconnection)
%
% Name: C.m
%
% Description: Flow set
%
% Version: 1.0
% Required files: - 
%%%%%%%%%%%%%%%%%%%%%%%%%%%%%%%%%%%%%%%%%%%%%%%%%%%%%%%%%%%%%%%%%%%%%%%%%%%

%flow set
if ((tau(2) >= 0) && (tau(2) < tau(3)))   % flow condition
    v = 1;  % report flow
else 
    v = 0;  % do not report flow
end

== matlab function Aperiodic Sampling 4/jump map g ==
  settings: updateMethod=DISCRETE
  data: tau input double; tauplus output double; u input double
function tauplus = g(tau, u)

%%%%%%%%%%%%%%%%%%%%%%%%%%%%%%%%%%%%%%%%%%%%%%%%%%%%%%%%%%%%%%%%%%%%%%%%%%%
% Matlab Function  Author: Ricardo Sanfelice 
%
% Project: Simulation of a hybrid system (interconnection)
%
% Name: g.m
%
% Description: Jump map
%
% Version: 1.0
% Required files: - 
%%%%%%%%%%%%%%%%%%%%%%%%%%%%%%%%%%%%%%%%%%%%%%%%%%%%%%%%%%%%%%%%%%%%%%%%%%%

% jump map
% if (1+e)*tau < 1
%     tauplus = (1+e)*tau;
% elseif (1+e)*tau >= 1
%     tauplus = 0;
% else
%     tauplus = tau;   
% end
tauplus = zeros(3,1);
tauplus(1) = u;
tauplus(2) = 0;
tauplus(3) = 0.3+0.35*rand;

== matlab function Aperiodic Sampling 4/jump set D ==
  data: tau input double; v output double; u input double
function v  = D(tau, u) 

%%%%%%%%%%%%%%%%%%%%%%%%%%%%%%%%%%%%%%%%%%%%%%%%%%%%%%%%%%%%%%%%%%%%%%%%%%%
% Matlab Function  Author: Ricardo Sanfelice
%
% Project: Simulation of a hybrid system (interconnection)
%
% Name: D.m
%
% Description: Jump set
%
% Version: 1.0
% Required files: - 
%%%%%%%%%%%%%%%%%%%%%%%%%%%%%%%%%%%%%%%%%%%%%%%%%%%%%%%%%%%%%%%%%%%%%%%%%%%

if (tau(2) >= tau(3)) % jump condition
    v = 1;  % report jump
else
    v = 0;  % do not report jump
end
